simulink model "mymodel"  (R2021b)
settings: Solver=VariableStepAuto  StartTime=0.0  StopTime=10.0  RelTol=1e-3
settings Model: Creator=Xavier  LastModifiedBy=Xavier

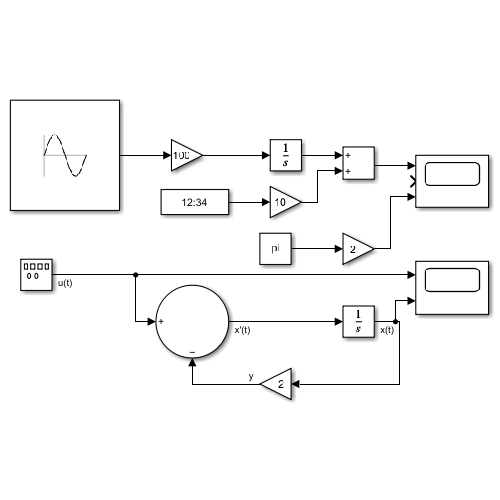
[thumbnail: Simulink's stored preview of the top-level diagram]
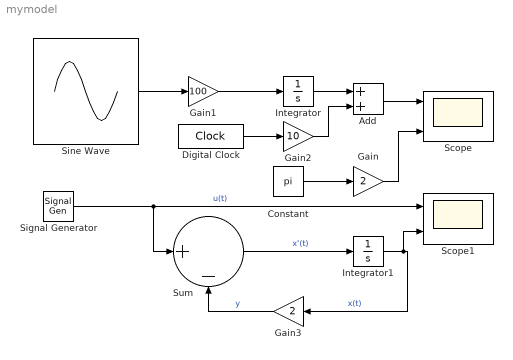
== system mymodel ==
  Add : Sum
  Constant : Constant  Value=pi
  Digital Clock : DigitalClock
  Gain : Gain  Gain=2
  Gain1 : Gain  Gain=100
  Gain2 : Gain  Gain=10
  Gain3 : Gain  Gain=2
  Integrator : Integrator
  Integrator1 : Integrator
  Scope : Scope  NumInputPorts=3
  Scope1 : Scope  NumInputPorts=2
  Signal Generator : SignalGenerator  WaveForm=random  Frequency=0.2
  Sine Wave : Sin  Frequency=50  SampleTime=0
  Sum : Sum  Inputs=|+-
  wires:
  Constant/1 -> Gain/1
  Digital Clock/1 -> Gain2/1
  Gain/1 -> Scope/3
  Gain3/1 -> Sum/2  "y"
  Gain2/1 -> Add/2
  Sine Wave/1 -> Gain1/1
  Sum/1 -> Integrator1/1  "x'(t)"
  Integrator/1 -> Add/1
  Gain1/1 -> Integrator/1
  Add/1 -> Scope/1
  Signal Generator/1 -> Sum/1, Scope1/1  "u(t)"
  Integrator1/1 -> Gain3/1, Scope1/2  "x(t)"
